simulink model "volumenpulmones"  (Simulink 7.5)
settings: Solver=ode45  StartTime=0.0  StopTime=10.0  RelTol=1e-3
settings Model: Creator=My Laptop  LastModifiedBy=My Laptop

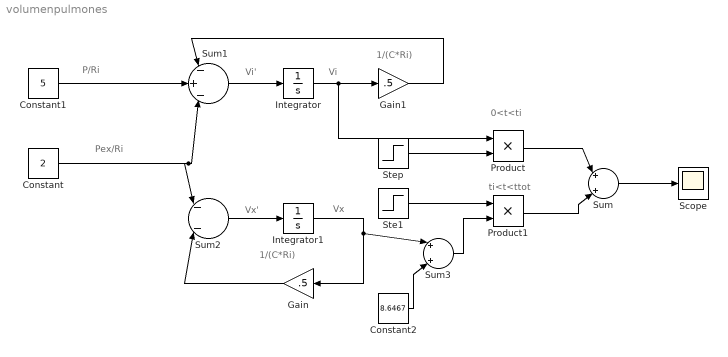
== system volumenpulmones ==
  note: Pex/Ri
  note: ti<t<ttot
  note: 0<t<ti
  note: P/Ri
  note: 1/(C*Ri)
  note: Vi'
  note: Vi
  note: Vx'
  note: Vx
  note: 1/(C*Ri)
  Constant : Constant  Value=2  OutDataType=fixdt(1, 16)  OutScaling=2^0
  Constant1 : Constant  Value=5  OutDataType=fixdt(1, 16)  OutScaling=2^0
  Constant2 : Constant  Value=8.6467  OutDataType=fixdt(1, 16)  OutScaling=2^0
  Gain : Gain  Gain=.5  ParameterDataType=fixdt(1, 16)  ParameterScaling=2^0  OutDataType=fixdt(1, 16)  OutScaling=2^0
  Gain1 : Gain  Gain=.5  ParameterDataType=fixdt(1, 16)  ParameterScaling=2^0  OutDataType=fixdt(1, 16)  OutScaling=2^0
  Integrator : Integrator
  Integrator1 : Integrator
  Product : Product  OutDataType=fixdt(1, 16)  OutScaling=2^0  RndMeth=Zero
  Product1 : Product  OutDataType=fixdt(1, 16)  OutScaling=2^0  RndMeth=Zero
  Scope : Scope
  Ste1 : Step  Time=4  SampleTime=0
  Step : Step  Time=4  Before=1  After=0  SampleTime=0
  Sum : Sum  Inputs=|+|+|  OutDataType=fixdt(1, 16)  OutScaling=2^0
  Sum1 : Sum  Inputs=|-|+|-|  OutDataType=fixdt(1, 16)  OutScaling=2^0
  Sum2 : Sum  Inputs=|-|-|  OutDataType=fixdt(1, 16)  OutScaling=2^0
  Sum3 : Sum  Inputs=|+|+|  OutDataType=fixdt(1, 16)  OutScaling=2^0
  wires:
  Sum/1 -> Scope/1
  Step/1 -> Product/2
  Sum1/1 -> Integrator/1
  Integrator/1 -> Gain1/1, Product/1
  Gain1/1 -> Sum1/1
  Constant/1 -> Sum1/3, Sum2/1
  Constant1/1 -> Sum1/2
  Ste1/1 -> Product1/1
  Sum2/1 -> Integrator1/1
  Integrator1/1 -> Sum3/1, Gain/1
  Gain/1 -> Sum2/2
  Product/1 -> Sum/1
  Product1/1 -> Sum/2
  Sum3/1 -> Product1/2
  Constant2/1 -> Sum3/2
